simulink model "TestPGR"  (R2023b)
settings: Solver=FixedStepAuto  StartTime=0.0  StopTime=inf  RelTol=1e-3  EnableMultiTasking=on
PreLoadFcn:
  | bool STATE = false;
model workspace (MAT data in the model file):
  Can_ID = 0
libraries: canmsglib x13, arduinolib x3
settings Model: ExtModeTrigDuration=2  Creator=Antonio  LastModifiedBy=Nuc1
settings OptimizationCC: EnhancedBackFolding=on  PassReuseOutputArgsAs=Individual arguments  ZeroExternalMemoryAtStartup=off  ZeroInternalMemoryAtStartup=off  MaxStackSize=64  OptimizeBlockOrder=speed  DifferentSizesBufferReuse=on  OptimizationCustomize=off  EfficientTunableParamExpr=on
settings DebuggingCC: ParameterTunabilityLossMsg=error
settings HardwareCC: ProdBitPerPointer=32  ProdBitPerSizeT=32  ProdBitPerPtrDiffT=32  ProdLargestAtomicInteger=Long  ProdLargestAtomicFloat=Double  ProdWordSize=32  ProdHWDeviceType=ARM Compatible->ARM Cortex
settings SFSimCC: MATLABDynamicMemAlloc=off
settings RTWCC: Description=Embedded Coder  SystemTargetFile=ert.tlc  HardwareBoard=Arduino MKR WiFi 1010  TemplateMakefile=ert_default_tmf  Toolchain=Arduino ARM  BuildConfiguration=Faster Runs
settings CodeAppCC: ForceParamTrailComments=on  IgnoreCustomStorageClasses=off  OperatorAnnotations=on  SimulinkDataObjDesc=on  SFDataObjDesc=on  InsertBlockDesc=on
settings ERTTargetCC: SupportContinuousTime=on  SupportVariableSizeSignals=on  ExtModeTransport=3  ExtModeStaticAlloc=on  ExtModeAutomaticAllocSize=off  ExtModeStaticAllocSize=8192  ExtModeMexFile=ext_xcp  ExtModeIntrfLevel=Level2 - Open

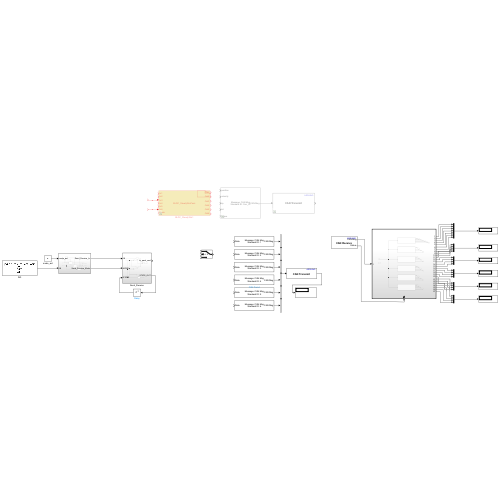
[thumbnail: Simulink's stored preview of the top-level diagram]
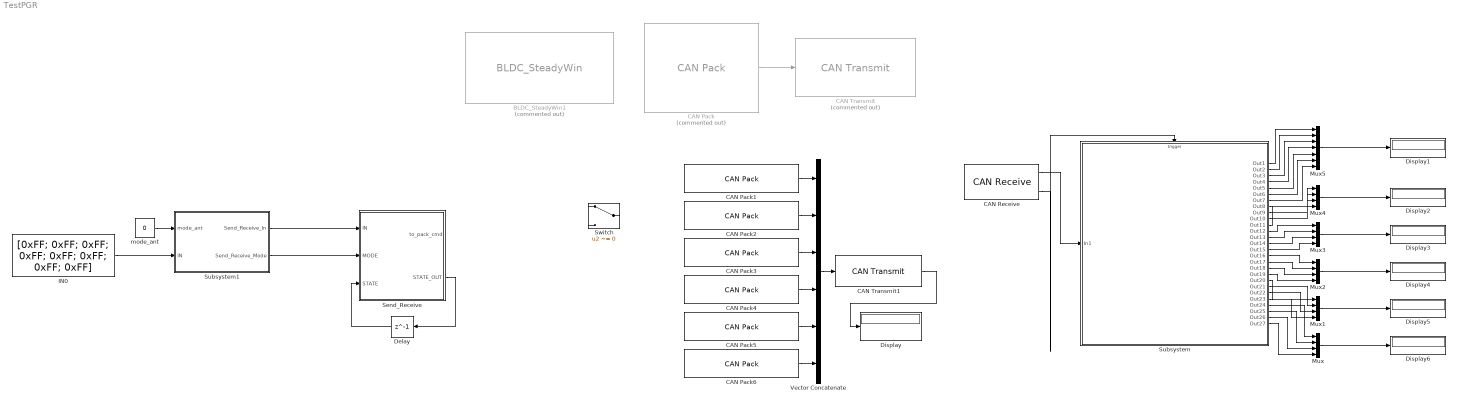
== system TestPGR ==
  BLDC_SteadyWin1 : S-Function  Commented=on  InitFcn=try, set_param(gcb,'FunctionName','BLDC_SteadyWin'), end  FunctionName=BLDC_SteadyWin  SFunctionModules=BLDC_SteadyWinPack_wrapper.cpp  SFunctionDeploymentMode=off  EnableBusSupport=off  mask(S-Function Builder){}
      mask help: Simulink:masks:SFunctionBuilder_MD
      mask init:
      | val = [[.9  0.75 0.75 1 1 .9 .9 1]',[1 1 0.75 0.75 .9 .9 1 .9]'];try , sys = get_param(gcb,'SfunBuilderFcnName');if isempty(sys), sys = get_param(gcb,'FunctionName'); end,catch, sys = get_param(gcb,'FunctionName'); end
      settings: CopyFcn=set_param(gcbh,'LinkStatus','none')  PreSaveFcn=try, set_param(gcb,'FunctionName','BLDC_SteadyWin'), end  OpenFcn=sfunctionwizard(gcbh)
      mask Display:
      | plot(val(:,1),val(:,2))
      | disp(sys)
      | port_label('input',1,'In1')
      | port_label('input',2,'In2')
      | port_label('input',3,'In3')
      | port_label('input',4,'In4')
      | port_label('input',5,'In5')
      | port_label('input',6,'In6')
      | port_label('input',7,'Mode')
      | port_label('output',1,'Out1')
      | port_label('output',2,'Out2')
      | port_label('output',3,'Out3')
      | port_label('output',4,'Out4')
      | port_label('output',5,'Out5')
      | port_label('output',6,'Out6')
  CAN Pack : canmsglib/CAN Pack  Commented=on  MsgList=(none)  MsgName=CAN Msg  MsgIDType=Standard (11-bit identifier)  MsgIdentifier=Can_ID  MsgLength=8  Remote=off  ApplyMinMax=off  BusOutput=off  SignalInfo={ 'position', '8', '16', 'BE', 'signed', 'Standard', '0', '1', '-95.5', '-95.5', '95.5'; 'velocity', '28', '12', 'BE', 'signed', 'Standard', '0', '1', '-45', '-45', '45'; 'kp', '32', '12', 'BE', 'unsigned', 'Standard', '0', '1', '0', '0', '500'; 'kd', '52', '12', 'BE', 'unsigned', 'Standard', '0', '1', '0', '0', '5'; 'torque', '56', '12', 'BE', 'signed', 'Standard', '0', '1', '-18', '-18', '18' }
      settings: LibrarySourceBlock=embeddedtargetslib/Host Communication/CAN Pack  DataFormat=manually specified signals
  CAN Pack1 : canmsglib/CAN Pack  MsgList=(none)  MsgName=CAN Msg  MsgIDType=Standard (11-bit identifier)  MsgIdentifier=1  MsgLength=8  Remote=off  ApplyMinMax=off  BusOutput=on  SignalInfo={ 'position', '8', '16', 'BE', 'signed', 'Standard', '0', '1', '-95.5', '-95.5', '95.5'; 'velocity', '28', '12', 'BE', 'signed', 'Standard', '0', '1', '-45', '-45', '45'; 'kp', '32', '12', 'BE', 'unsigned', 'Standard', '0', '1', '0', '0', '500'; 'kd', '52', '12', 'BE', 'unsigned', 'Standard', '0', '1', '0', '0', '5'; 'torque', '56', '12', 'BE', 'signed', 'Standard', '0', '1', '-18', '-18', '18' }
      settings: LibrarySourceBlock=embeddedtargetslib/Host Communication/CAN Pack  DataFormat=raw data
  CAN Pack2 : canmsglib/CAN Pack  MsgList=(none)  MsgName=CAN Msg  MsgIDType=Standard (11-bit identifier)  MsgIdentifier=2  MsgLength=8  Remote=off  ApplyMinMax=off  BusOutput=on  SignalInfo={ 'position', '8', '16', 'BE', 'signed', 'Standard', '0', '1', '-95.5', '-95.5', '95.5'; 'velocity', '28', '12', 'BE', 'signed', 'Standard', '0', '1', '-45', '-45', '45'; 'kp', '32', '12', 'BE', 'unsigned', 'Standard', '0', '1', '0', '0', '500'; 'kd', '52', '12', 'BE', 'unsigned', 'Standard', '0', '1', '0', '0', '5'; 'torque', '56', '12', 'BE', 'signed', 'Standard', '0', '1', '-18', '-18', '18' }
      settings: LibrarySourceBlock=embeddedtargetslib/Host Communication/CAN Pack  DataFormat=raw data
  CAN Pack3 : canmsglib/CAN Pack  MsgList=(none)  MsgName=CAN Msg  MsgIDType=Standard (11-bit identifier)  MsgIdentifier=3  MsgLength=8  Remote=off  ApplyMinMax=off  BusOutput=on  SignalInfo={ 'position', '8', '16', 'BE', 'signed', 'Standard', '0', '1', '-95.5', '-95.5', '95.5'; 'velocity', '28', '12', 'BE', 'signed', 'Standard', '0', '1', '-45', '-45', '45'; 'kp', '32', '12', 'BE', 'unsigned', 'Standard', '0', '1', '0', '0', '500'; 'kd', '52', '12', 'BE', 'unsigned', 'Standard', '0', '1', '0', '0', '5'; 'torque', '56', '12', 'BE', 'signed', 'Standard', '0', '1', '-18', '-18', '18' }
      settings: LibrarySourceBlock=embeddedtargetslib/Host Communication/CAN Pack  DataFormat=raw data
  CAN Pack4 : canmsglib/CAN Pack  MsgList=(none)  MsgName=CAN Msg  MsgIDType=Standard (11-bit identifier)  MsgIdentifier=4  MsgLength=8  Remote=off  ApplyMinMax=off  BusOutput=on  SignalInfo={ 'position', '8', '16', 'BE', 'signed', 'Standard', '0', '1', '-95.5', '-95.5', '95.5'; 'velocity', '28', '12', 'BE', 'signed', 'Standard', '0', '1', '-45', '-45', '45'; 'kp', '32', '12', 'BE', 'unsigned', 'Standard', '0', '1', '0', '0', '500'; 'kd', '52', '12', 'BE', 'unsigned', 'Standard', '0', '1', '0', '0', '5'; 'torque', '56', '12', 'BE', 'signed', 'Standard', '0', '1', '-18', '-18', '18' }
      settings: LibrarySourceBlock=embeddedtargetslib/Host Communication/CAN Pack  DataFormat=raw data
  CAN Pack5 : canmsglib/CAN Pack  MsgList=(none)  MsgName=CAN Msg  MsgIDType=Standard (11-bit identifier)  MsgIdentifier=5  MsgLength=8  Remote=off  ApplyMinMax=off  BusOutput=on  SignalInfo={ 'position', '8', '16', 'BE', 'signed', 'Standard', '0', '1', '-95.5', '-95.5', '95.5'; 'velocity', '28', '12', 'BE', 'signed', 'Standard', '0', '1', '-45', '-45', '45'; 'kp', '32', '12', 'BE', 'unsigned', 'Standard', '0', '1', '0', '0', '500'; 'kd', '52', '12', 'BE', 'unsigned', 'Standard', '0', '1', '0', '0', '5'; 'torque', '56', '12', 'BE', 'signed', 'Standard', '0', '1', '-18', '-18', '18' }
      settings: LibrarySourceBlock=embeddedtargetslib/Host Communication/CAN Pack  DataFormat=raw data
  CAN Pack6 : canmsglib/CAN Pack  MsgList=(none)  MsgName=CAN Msg  MsgIDType=Standard (11-bit identifier)  MsgIdentifier=6  MsgLength=8  Remote=off  ApplyMinMax=off  BusOutput=on  SignalInfo={ 'position', '8', '16', 'BE', 'signed', 'Standard', '0', '1', '-95.5', '-95.5', '95.5'; 'velocity', '28', '12', 'BE', 'signed', 'Standard', '0', '1', '-45', '-45', '45'; 'kp', '32', '12', 'BE', 'unsigned', 'Standard', '0', '1', '0', '0', '500'; 'kd', '52', '12', 'BE', 'unsigned', 'Standard', '0', '1', '0', '0', '5'; 'torque', '56', '12', 'BE', 'signed', 'Standard', '0', '1', '-18', '-18', '18' }
      settings: LibrarySourceBlock=embeddedtargetslib/Host Communication/CAN Pack  DataFormat=raw data
  CAN Receive : arduinolib/CAN Receive  outputDataType=CAN Msg  identifierType=Standard (11-bit identifier)  messageId=100  msgLength=8  SampleTime=0.1  outputError=off  outputRemote=off
  CAN Transmit : arduinolib/CAN Transmit  Commented=on  inputDataType=CAN Msg  BlockingMode_=on  BlockTimeout_=1  outputStatus=on  identifierType=Standard (11-bit identifier)  messageId=100  msgLength=8  remoteFrame=off
  CAN Transmit1 : arduinolib/CAN Transmit  inputDataType=CAN Msg  BlockingMode_=on  BlockTimeout_=1  outputStatus=on  identifierType=Standard (11-bit identifier)  messageId=100  msgLength=8  remoteFrame=off
  Delay : Delay  DelayLength=1  StateName=STATE
  Display{,1..6} (7 alike) : Display
  IN0 : Constant  Value=|  OutDataTypeStr=uint8
      | [0xFF; 0xFF; 0xFF; 0xFF; 0xFF;
      | 0xFF;
      | 0xFF;
      | 0xFF]
  Mux{,1..4} (5 alike) : Mux
  Mux5 : Mux  Inputs=7
  Send_Receive : Subsystem
  Subsystem : Subsystem
  Subsystem1 : Subsystem
  Switch : Switch  Criteria=u2 ~= 0  SaturateOnIntegerOverflow=off  InputSameDT=off
  Vector Concatenate : Concatenate  NumInputs=6
  mode_ant : Constant  Value=0
  wires:
  CAN Pack/1 -> CAN Transmit/1
  CAN Transmit1/1 -> Display/1
  CAN Receive/1 -> Subsystem/1(In1)
  CAN Receive/2 -> Subsystem/Trigger
  CAN Pack1/1 -> Vector Concatenate/1
  CAN Pack2/1 -> Vector Concatenate/2
  CAN Pack3/1 -> Vector Concatenate/3
  CAN Pack4/1 -> Vector Concatenate/4
  CAN Pack5/1 -> Vector Concatenate/5
  CAN Pack6/1 -> Vector Concatenate/6
  Vector Concatenate/1 -> CAN Transmit1/1
  Subsystem/25(Out25) -> Mux/2
  Subsystem/24(Out24) -> Mux/1
  Subsystem/26(Out26) -> Mux/3
  Subsystem/27(Out27) -> Mux/4
  Subsystem/20(Out20) -> Mux1/1
  Subsystem/21(Out21) -> Mux1/2
  Subsystem/22(Out22) -> Mux1/3
  Subsystem/23(Out23) -> Mux1/4
  Subsystem/16(Out16) -> Mux2/1
  Subsystem/17(Out17) -> Mux2/2
  Subsystem/18(Out18) -> Mux2/3
  Subsystem/19(Out19) -> Mux2/4
  Subsystem/12(Out12) -> Mux3/1
  Subsystem/13(Out13) -> Mux3/2
  Subsystem/14(Out14) -> Mux3/3
  Subsystem/15(Out15) -> Mux3/4
  Subsystem/10(Out10) -> Mux4/3
  Subsystem/9(Out9) -> Mux4/2
  Subsystem/8(Out8) -> Mux4/1
  Subsystem/11(Out11) -> Mux4/4
  Subsystem/1(Out1) -> Mux5/1
  Subsystem/2(Out2) -> Mux5/2
  Subsystem/3(Out3) -> Mux5/3
  Subsystem/4(Out4) -> Mux5/4
  Subsystem/5(Out5) -> Mux5/5
  Subsystem/6(Out6) -> Mux5/6
  Subsystem/7(Out7) -> Mux5/7
  Mux5/1 -> Display1/1
  Mux4/1 -> Display2/1
  Mux3/1 -> Display3/1
  Mux2/1 -> Display4/1
  Mux1/1 -> Display5/1
  Mux/1 -> Display6/1
  ? -> BLDC_SteadyWin1/3
  ? -> BLDC_SteadyWin1/6
  Subsystem1/2(Send_Receive_Mode) -> Send_Receive/2(MODE)
  Subsystem1/1(Send_Receive_In) -> Send_Receive/1(IN)
  Send_Receive/2(STATE_OUT) -> Delay/1
  Delay/1 -> Send_Receive/3(STATE)
  mode_ant/1 -> Subsystem1/1(mode_ant)
  IN0/1 -> Subsystem1/2(IN)

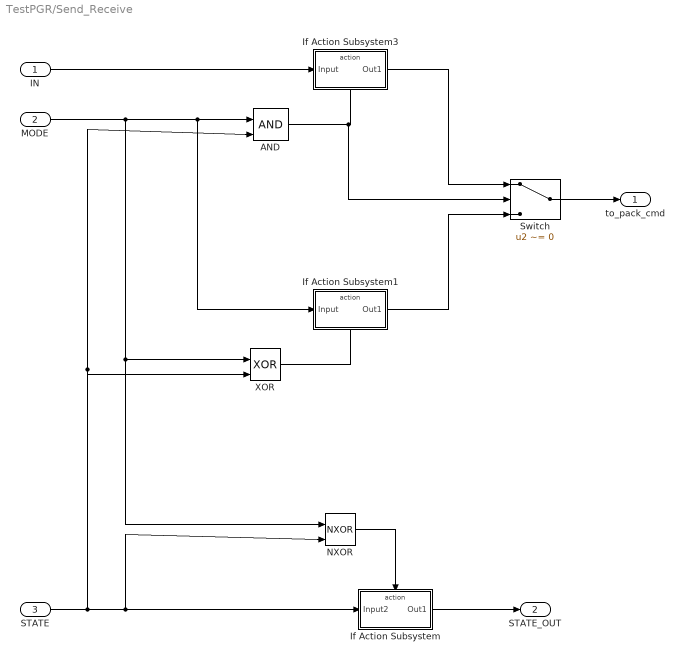
== system TestPGR/Send_Receive ==
  IN : Inport
  MODE : Inport  Port=2
  STATE : Inport  Port=3
  AND : Logic  IconShape=distinctive  AllPortsSameDT=off  OutDataTypeStr=boolean
  If Action Subsystem : Subsystem  TreatAsAtomicUnit=on
  If Action Subsystem1 : Subsystem  TreatAsAtomicUnit=on
  If Action Subsystem3 : Subsystem  TreatAsAtomicUnit=on
  NXOR : Logic  Operator=NXOR  IconShape=distinctive  AllPortsSameDT=off  OutDataTypeStr=boolean
  Switch : Switch  Criteria=u2 ~= 0  SaturateOnIntegerOverflow=off  InputSameDT=off
  XOR : Logic  Operator=XOR  IconShape=distinctive  AllPortsSameDT=off  OutDataTypeStr=boolean
  to_pack_cmd : Outport
  STATE_OUT : Outport  Port=2
  wires:
  STATE/1 -> AND/2, XOR/2, NXOR/2, If Action Subsystem/1(Input2)
  NXOR/1 -> If Action Subsystem/Action
  If Action Subsystem/1(Out1) -> STATE_OUT/1
  IN/1 -> If Action Subsystem3/1(Input)
  AND/1 -> Switch/2, If Action Subsystem3/Action
  MODE/1 -> NXOR/1, XOR/1, If Action Subsystem1/1(Input), AND/1
  XOR/1 -> If Action Subsystem1/Action
  If Action Subsystem3/1(Out1) -> Switch/1
  If Action Subsystem1/1(Out1) -> Switch/3
  Switch/1 -> to_pack_cmd/1

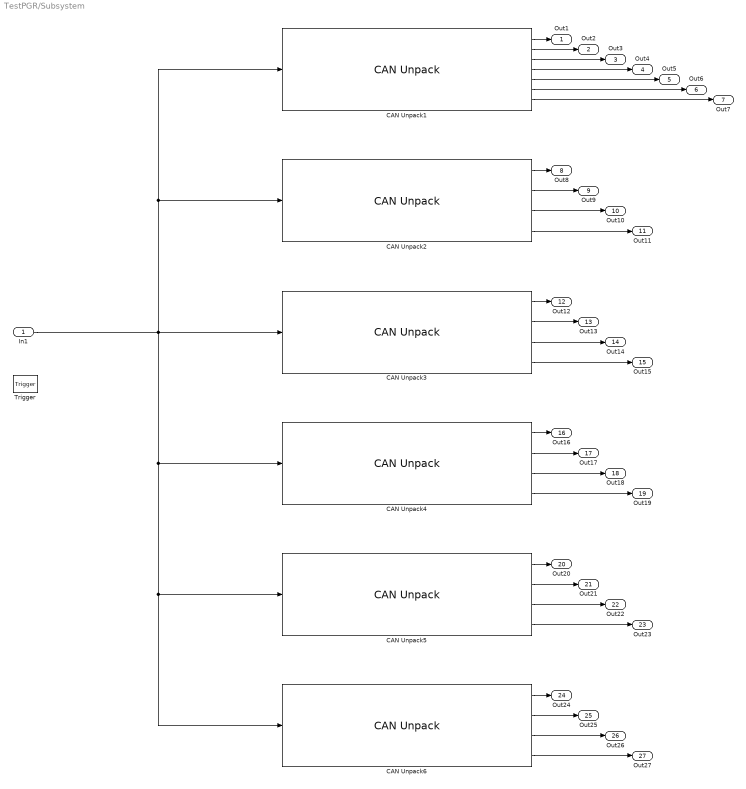
== system TestPGR/Subsystem ==
  In1 : Inport
  Trigger : TriggerPort  VariantControl=(inherit)  PortDimensions=1
  CAN Unpack1 : canmsglib/CAN Unpack  MsgList=(none)  MsgName=CAN Msg  MsgIDType=Standard (11-bit identifier)  MsgIdentifier=1  MsgLength=5  SignalInfo={ 'position', '8', '16', 'BE', 'signed', 'Standard', '0', '343.11518324607329842931937172775', '-95.5', '-95.5', '95.5'; 'velocity', '28', '12', 'BE', 'signed', 'Standard', '0', '45.5', '-45', '-45', '45'; 'current', '32', '12', 'BE', 'signed', 'Standard', '0', '113.75', '-18', '-18', '18' }  IDPort=on  TimestampPort=on  ErrorPort=on  RemotePort=off  LengthPort=off  StatusPort=on  ApplyMinMax=off
      settings: LibrarySourceBlock=embeddedtargetslib/Host Communication/CAN Unpack
  CAN Unpack2 : canmsglib/CAN Unpack  MsgList=(none)  MsgName=CAN Msg  MsgIDType=Standard (11-bit identifier)  MsgIdentifier=2  MsgLength=5  SignalInfo={ 'position', '8', '16', 'BE', 'signed', 'Standard', '0', '343.11518324607329842931937172775', '-95.5', '-95.5', '95.5'; 'velocity', '28', '12', 'BE', 'signed', 'Standard', '0', '45.5', '-45', '-45', '45'; 'current', '32', '12', 'BE', 'signed', 'Standard', '0', '113.75', '-18', '-18', '18' }  IDPort=on  TimestampPort=off  ErrorPort=off  RemotePort=off  LengthPort=off  StatusPort=off  ApplyMinMax=off
      settings: LibrarySourceBlock=embeddedtargetslib/Host Communication/CAN Unpack
  CAN Unpack3 : canmsglib/CAN Unpack  MsgList=(none)  MsgName=CAN Msg  MsgIDType=Standard (11-bit identifier)  MsgIdentifier=3  MsgLength=5  SignalInfo={ 'position', '8', '16', 'BE', 'signed', 'Standard', '0', '343.11518324607329842931937172775', '-95.5', '-95.5', '95.5'; 'velocity', '28', '12', 'BE', 'signed', 'Standard', '0', '45.5', '-45', '-45', '45'; 'current', '32', '12', 'BE', 'signed', 'Standard', '0', '113.75', '-18', '-18', '18' }  IDPort=on  TimestampPort=off  ErrorPort=off  RemotePort=off  LengthPort=off  StatusPort=off  ApplyMinMax=off
      settings: LibrarySourceBlock=embeddedtargetslib/Host Communication/CAN Unpack
  CAN Unpack4 : canmsglib/CAN Unpack  MsgList=(none)  MsgName=CAN Msg  MsgIDType=Standard (11-bit identifier)  MsgIdentifier=4  MsgLength=5  SignalInfo={ 'position', '8', '16', 'BE', 'signed', 'Standard', '0', '343.11518324607329842931937172775', '-95.5', '-95.5', '95.5'; 'velocity', '28', '12', 'BE', 'signed', 'Standard', '0', '45.5', '-45', '-45', '45'; 'current', '32', '12', 'BE', 'signed', 'Standard', '0', '113.75', '-18', '-18', '18' }  IDPort=on  TimestampPort=off  ErrorPort=off  RemotePort=off  LengthPort=off  StatusPort=off  ApplyMinMax=off
      settings: LibrarySourceBlock=embeddedtargetslib/Host Communication/CAN Unpack
  CAN Unpack5 : canmsglib/CAN Unpack  MsgList=(none)  MsgName=CAN Msg  MsgIDType=Standard (11-bit identifier)  MsgIdentifier=5  MsgLength=5  SignalInfo={ 'position', '8', '16', 'BE', 'signed', 'Standard', '0', '343.11518324607329842931937172775', '-95.5', '-95.5', '95.5'; 'velocity', '28', '12', 'BE', 'signed', 'Standard', '0', '45.5', '-45', '-45', '45'; 'current', '32', '12', 'BE', 'signed', 'Standard', '0', '113.75', '-18', '-18', '18' }  IDPort=on  TimestampPort=off  ErrorPort=off  RemotePort=off  LengthPort=off  StatusPort=off  ApplyMinMax=off
      settings: LibrarySourceBlock=embeddedtargetslib/Host Communication/CAN Unpack
  CAN Unpack6 : canmsglib/CAN Unpack  MsgList=(none)  MsgName=CAN Msg  MsgIDType=Standard (11-bit identifier)  MsgIdentifier=6  MsgLength=5  SignalInfo={ 'position', '8', '16', 'BE', 'signed', 'Standard', '0', '343.11518324607329842931937172775', '-95.5', '-95.5', '95.5'; 'velocity', '28', '12', 'BE', 'signed', 'Standard', '0', '45.5', '-45', '-45', '45'; 'current', '32', '12', 'BE', 'signed', 'Standard', '0', '113.75', '-18', '-18', '18' }  IDPort=on  TimestampPort=off  ErrorPort=off  RemotePort=off  LengthPort=off  StatusPort=off  ApplyMinMax=off
      settings: LibrarySourceBlock=embeddedtargetslib/Host Communication/CAN Unpack
  Out1 : Outport
  Out2 : Outport  Port=2
  Out3 : Outport  Port=3
  Out4 : Outport  Port=4
  Out5 : Outport  Port=5
  Out6 : Outport  Port=6
  Out7 : Outport  Port=7
  Out8 : Outport  Port=8
  Out9 : Outport  Port=9
  Out10 : Outport  Port=10
  Out11 : Outport  Port=11
  Out12 : Outport  Port=12
  Out13 : Outport  Port=13
  Out14 : Outport  Port=14
  Out15 : Outport  Port=15
  Out16 : Outport  Port=16
  Out17 : Outport  Port=17
  Out18 : Outport  Port=18
  Out19 : Outport  Port=19
  Out20 : Outport  Port=20
  Out21 : Outport  Port=21
  Out22 : Outport  Port=22
  Out23 : Outport  Port=23
  Out24 : Outport  Port=24
  Out25 : Outport  Port=25
  Out26 : Outport  Port=26
  Out27 : Outport  Port=27
  wires:
  CAN Unpack1/2 -> Out2/1
  CAN Unpack1/7 -> Out7/1
  CAN Unpack1/5 -> Out5/1
  CAN Unpack1/4 -> Out4/1
  CAN Unpack1/1 -> Out1/1
  CAN Unpack1/6 -> Out6/1
  CAN Unpack1/3 -> Out3/1
  In1/1 -> CAN Unpack6/1, CAN Unpack5/1, CAN Unpack4/1, CAN Unpack1/1, CAN Unpack2/1, CAN Unpack3/1
  CAN Unpack2/1 -> Out8/1
  CAN Unpack2/2 -> Out9/1
  CAN Unpack2/3 -> Out10/1
  CAN Unpack2/4 -> Out11/1
  CAN Unpack3/2 -> Out13/1
  CAN Unpack3/4 -> Out15/1
  CAN Unpack3/3 -> Out14/1
  CAN Unpack3/1 -> Out12/1
  CAN Unpack4/1 -> Out16/1
  CAN Unpack4/3 -> Out18/1
  CAN Unpack4/4 -> Out19/1
  CAN Unpack4/2 -> Out17/1
  CAN Unpack5/2 -> Out21/1
  CAN Unpack5/4 -> Out23/1
  CAN Unpack5/3 -> Out22/1
  CAN Unpack5/1 -> Out20/1
  CAN Unpack6/1 -> Out24/1
  CAN Unpack6/3 -> Out26/1
  CAN Unpack6/4 -> Out27/1
  CAN Unpack6/2 -> Out25/1

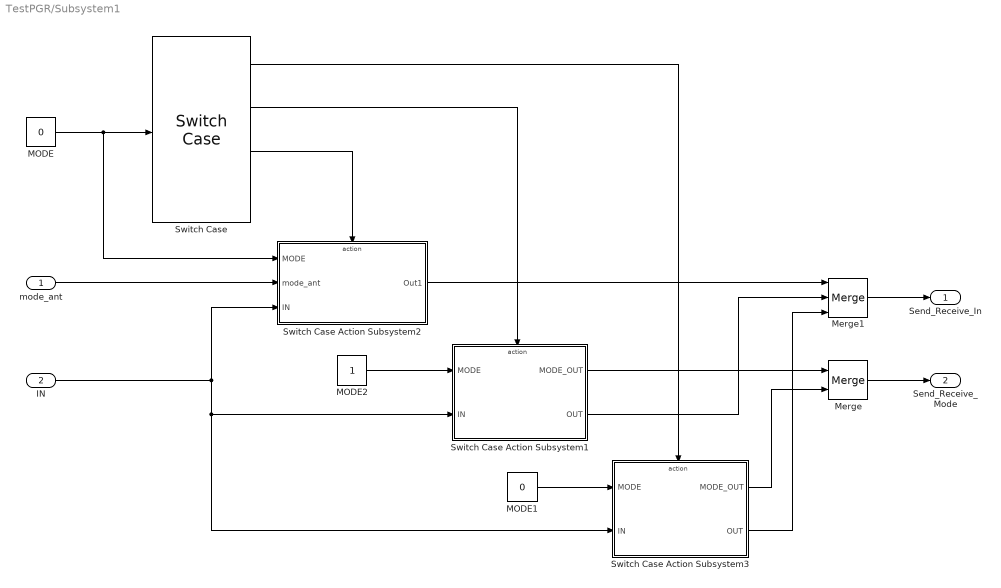
== system TestPGR/Subsystem1 ==
  mode_ant : Inport
  IN : Inport  Port=2
  MODE : Constant  Value=0
  MODE1 : Constant  Value=0
  MODE2 : Constant
  Merge : Merge
  Merge1 : Merge  Inputs=3
  Switch Case : SwitchCase  CaseConditions={0 1 2}
  Switch Case Action Subsystem1 : Subsystem  TreatAsAtomicUnit=on
  Switch Case Action Subsystem2 : Subsystem  TreatAsAtomicUnit=on
  Switch Case Action Subsystem3 : Subsystem  TreatAsAtomicUnit=on
  Send_Receive_In : Outport
  Send_Receive_Mode : Outport  Port=2
  wires:
  MODE/1 -> Switch Case Action Subsystem2/1(MODE), Switch Case/1
  Switch Case/1 -> Switch Case Action Subsystem3/Action
  MODE1/1 -> Switch Case Action Subsystem3/1(MODE)
  Switch Case/2 -> Switch Case Action Subsystem1/Action
  Switch Case/3 -> Switch Case Action Subsystem2/Action
  MODE2/1 -> Switch Case Action Subsystem1/1(MODE)
  mode_ant/1 -> Switch Case Action Subsystem2/2(mode_ant)
  IN/1 -> Switch Case Action Subsystem3/2(IN), Switch Case Action Subsystem1/2(IN), Switch Case Action Subsystem2/3(IN)
  Merge/1 -> Send_Receive_Mode/1
  Switch Case Action Subsystem3/1(MODE_OUT) -> Merge/2
  Switch Case Action Subsystem1/1(MODE_OUT) -> Merge/1
  Switch Case Action Subsystem2/1(Out1) -> Merge1/1
  Switch Case Action Subsystem1/2(OUT) -> Merge1/2
  Switch Case Action Subsystem3/2(OUT) -> Merge1/3
  Merge1/1 -> Send_Receive_In/1

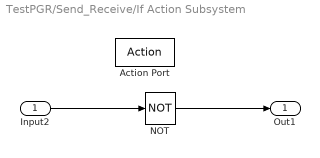
== system TestPGR/Send_Receive/If Action Subsystem ==
  Input2 : Inport
  Action Port : ActionPort
  NOT : Logic  Operator=NOT  IconShape=distinctive  AllPortsSameDT=off  OutDataTypeStr=boolean
  Out1 : Outport
  wires:
  Input2/1 -> NOT/1
  NOT/1 -> Out1/1

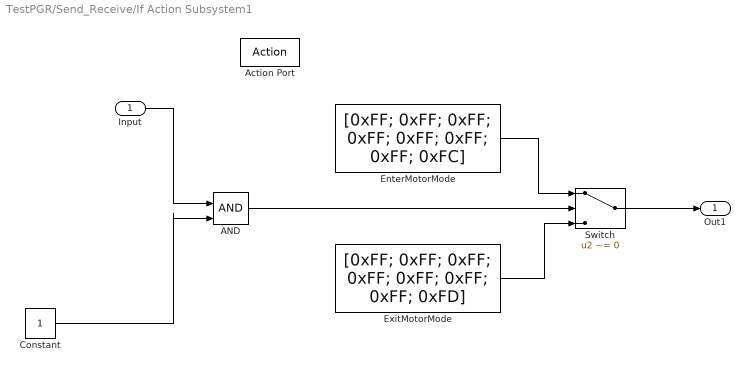
== system TestPGR/Send_Receive/If Action Subsystem1 ==
  Input : Inport
  Action Port : ActionPort
  AND : Logic  IconShape=distinctive  AllPortsSameDT=off  OutDataTypeStr=boolean
  Constant : Constant
  EnterMotorMode : Constant  Value=|  OutDataTypeStr=uint8
      | [0xFF; 0xFF; 0xFF; 0xFF; 0xFF;
      | 0xFF;
      | 0xFF;
      | 0xFC]
  ExitMotorMode : Constant  Value=|  OutDataTypeStr=uint8
      | [0xFF; 0xFF; 0xFF; 0xFF; 0xFF;
      | 0xFF;
      | 0xFF;
      | 0xFD]
  Switch : Switch  Criteria=u2 ~= 0  SaturateOnIntegerOverflow=off  InputSameDT=off
  Out1 : Outport
  wires:
  Input/1 -> AND/1
  Constant/1 -> AND/2
  AND/1 -> Switch/2
  EnterMotorMode/1 -> Switch/1
  Switch/1 -> Out1/1
  ExitMotorMode/1 -> Switch/3

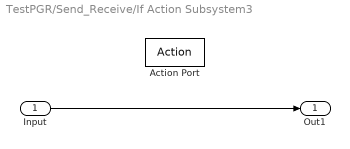
== system TestPGR/Send_Receive/If Action Subsystem3 ==
  Input : Inport
  Action Port : ActionPort
  Out1 : Outport
  wires:
  Input/1 -> Out1/1

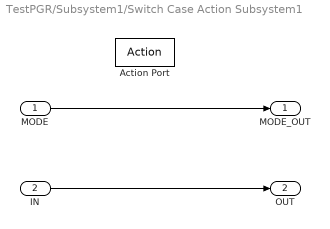
== system TestPGR/Subsystem1/Switch Case Action Subsystem1 ==
  MODE : Inport
  IN : Inport  Port=2
  Action Port : ActionPort  ActionPortLabel=case [ 1 ]:
  MODE_OUT : Outport
  OUT : Outport  Port=2
  wires:
  MODE/1 -> MODE_OUT/1
  IN/1 -> OUT/1

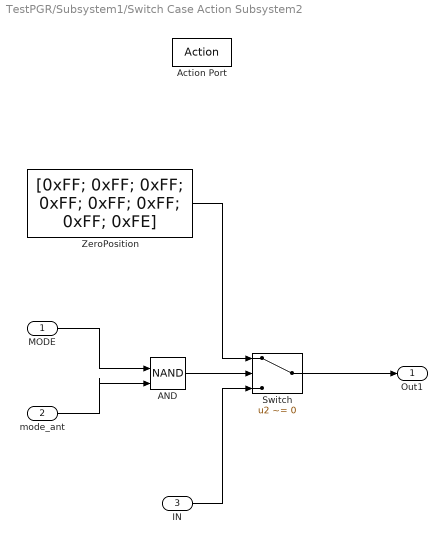
== system TestPGR/Subsystem1/Switch Case Action Subsystem2 ==
  MODE : Inport
  mode_ant : Inport  Port=2
  IN : Inport  Port=3
  Action Port : ActionPort  ActionPortLabel=case [ 2 ]:
  AND : Logic  Operator=NAND  IconShape=distinctive  AllPortsSameDT=off  OutDataTypeStr=boolean
  Switch : Switch  Criteria=u2 ~= 0  SaturateOnIntegerOverflow=off  InputSameDT=off
  ZeroPosition : Constant  Value=|  OutDataTypeStr=uint8
      | [0xFF; 0xFF; 0xFF; 0xFF; 0xFF;
      | 0xFF;
      | 0xFF;
      | 0xFE]
  Out1 : Outport
  wires:
  MODE/1 -> AND/1
  mode_ant/1 -> AND/2
  ZeroPosition/1 -> Switch/1
  AND/1 -> Switch/2
  Switch/1 -> Out1/1
  IN/1 -> Switch/3

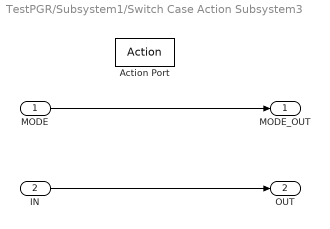
== system TestPGR/Subsystem1/Switch Case Action Subsystem3 ==
  MODE : Inport
  IN : Inport  Port=2
  Action Port : ActionPort  ActionPortLabel=case [ 0 ]:
  MODE_OUT : Outport
  OUT : Outport  Port=2
  wires:
  MODE/1 -> MODE_OUT/1
  IN/1 -> OUT/1
